simulink model "inner_LQRI_test"  (R2016a)
settings: Solver=VariableStepAuto  StartTime=0.0  StopTime=60  RelTol=1e-3
undefined symbols (not defined in the file or in its folder): b, g, inner_h, inner_maxlim, inner_minlim, K, k, l, m, max_ang_ref
settings Model: Creator=Daniel  LastModifiedBy=mgreiff
settings SolverCC: AlgebraicLoopSolver=LineSearch
settings DataIOCC: LimitDataPoints=on
settings DebuggingCC: AllowSymbolicDim=off
settings ModelReferenceCC: PropagateSignalLabelsOutOfModel=off
settings GRTTargetCC: GeneratePreprocessorConditionals=Use local settings

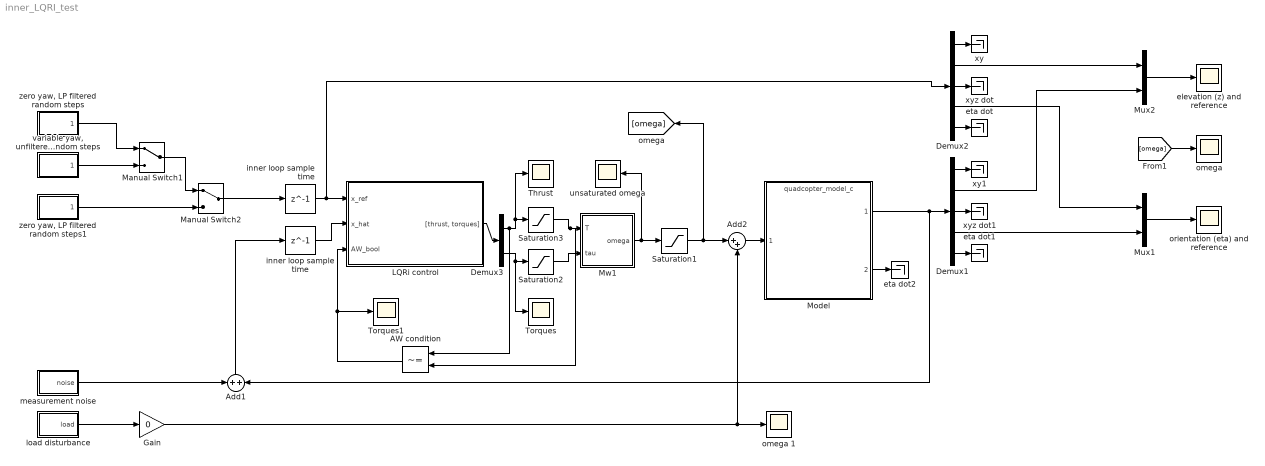
== system inner_LQRI_test ==
  "   eta dot" : Terminator
  "   eta dot1" : Terminator
  "   eta dot2" : Terminator
  "   xy" : Terminator
  "   xy1" : Terminator
  "  xyz dot" : Terminator
  "  xyz dot1" : Terminator
  AW condition : RelationalOperator  Operator=~=  OutDataTypeStr=boolean
  Add1 : Sum
  Add2 : Sum  Inputs=|++
  Demux1 : Demux  Outputs=[2,1,3,3,3]
  Demux2 : Demux  Outputs=[2,1,3,3,3]
  Demux3 : Demux  Outputs=[1,3]
  Gain : Gain  Gain=0
  LQRi control : Subsystem
  Manual Switch1 : ManualSwitch
  Manual Switch2 : ManualSwitch
  Model : ModelReference  ModelNameDialog=quadcopter_model_c.mdl  SimulationMode=Normal  ModelReferenceVersion=1.156
  Mux1 : Mux  Inputs=2
  Mux2 : Mux  Inputs=2
  Mw1 : Subsystem
  Saturation1 : Saturate  UpperLimit=inner_maxlim  LowerLimit=inner_minlim
  Saturation2 : Saturate  UpperLimit=0.1  LowerLimit=-0.1
  Saturation3 : Saturate  LowerLimit=0.01
  Thrust : Scope
  Torques : Scope
  Torques1 : Scope
  elevation (z) and reference : Scope
  inner loop sample time : Delay  DelayLength=1  InitialCondition=0  SampleTime=inner_h
  "inner loop sample time " : Delay  DelayLength=1  InitialCondition=0  SampleTime=inner_h
  load disturbance : Subsystem
  measurement noise : Subsystem
  "omega " : Scope
  omega 1 : Scope
  orientation (eta) and reference : Scope
  unsaturated omega : Scope
  "variable yaw, unfiltered random steps" : Subsystem
  "zero yaw, LP filtered random steps" : Subsystem
  "zero yaw, LP filtered random steps1" : Subsystem
  wires:
  Demux2/2 -> Mux2/1
  Mux2/1 -> elevation (z) and reference/1
  Demux1/2 -> Mux2/2
  Model/1 -> Demux1/1, Add1/2
  Mux1/1 -> orientation (eta) and reference/1
  Saturation1/1 -> [omega], Add2/1
  "inner loop sample time "/1 -> LQRi control/2(x_hat)
  Demux2/3 -> "  xyz dot"/1
  Demux2/5 -> "   eta dot"/1
  Demux2/1 -> "   xy"/1
  Demux1/3 -> "  xyz dot1"/1
  Demux1/5 -> "   eta dot1"/1
  Demux1/1 -> "   xy1"/1
  Demux1/4 -> Mux1/2
  [omega] -> "omega "/1
  Model/2 -> "   eta dot2"/1
  Demux2/4 -> Mux1/1
  AW condition/1 -> Torques1/1, LQRi control/3(AW_bool)
  inner loop sample time/1 -> LQRi control/1(x_ref), Demux2/1
  Manual Switch2/1 -> inner loop sample time/1
  load disturbance/1(load) -> Gain/1
  measurement noise/1(noise) -> Add1/1
  Manual Switch1/1 -> Manual Switch2/1
  Add1/1 -> "inner loop sample time "/1
  Add2/1 -> Model/1
  LQRi control/1("[thrust, torques]") -> Demux3/1
  Demux3/1 -> AW condition/1, Thrust/1, Saturation3/1
  Demux3/2 -> Torques/1, Saturation2/1
  Mw1/1(omega) -> unsaturated omega/1, Saturation1/1
  Saturation2/1 -> Mw1/2(tau)
  Saturation3/1 -> AW condition/2, Mw1/1(T)
  "variable yaw, unfiltered random steps"/1(reference) -> Manual Switch1/2
  "zero yaw, LP filtered random steps"/1(reference) -> Manual Switch1/1
  "zero yaw, LP filtered random steps1"/1(reference) -> Manual Switch2/2
  Gain/1 -> Add2/2, omega 1/1

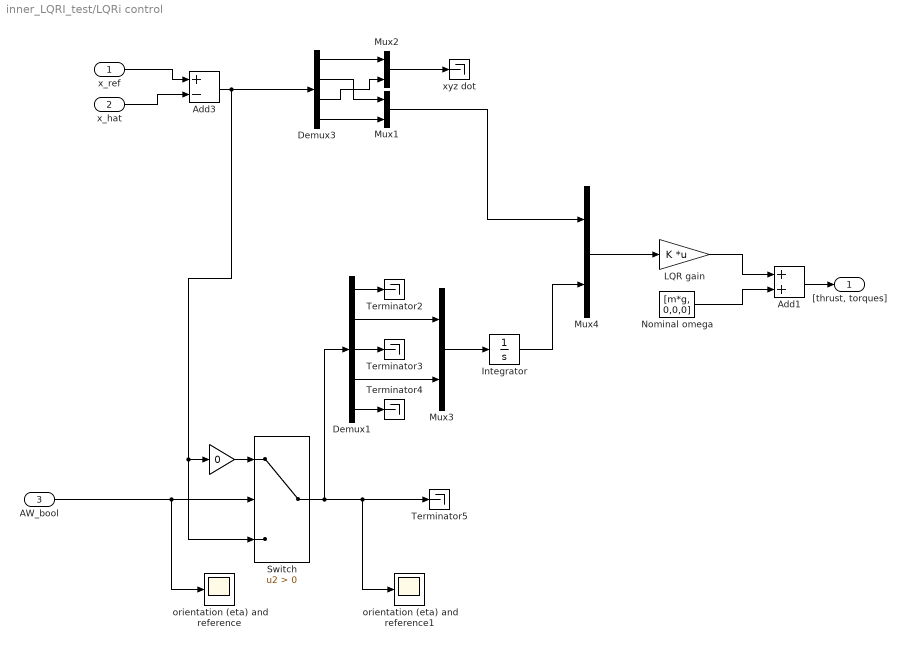
== system inner_LQRI_test/LQRi control ==
  x_ref : Inport  PortDimensions=12
  x_hat : Inport  Port=2  PortDimensions=12
  AW_bool : Inport  Port=3  PortDimensions=1
  "    " : Gain  Gain=0
  "  xyz dot" : Terminator
  Add1 : Sum
  Add3 : Sum  Inputs=+-
  Demux1 : Demux  Outputs=[2,1,3,3,3]
  Demux3 : Demux  Outputs=[2,1,2,7]
  Integrator : Integrator
  LQR gain : Gain  Gain=K  Multiplication=Matrix(K*u)
  Mux{1..4} (4 alike) : Mux  Inputs=2
  Nominal omega : Constant  Value=[m*g, 0,0,0]
  Switch : Switch  Criteria=u2 > Threshold
  Terminator{2..5} (4 alike) : Terminator
  orientation (eta) and reference : Scope
  orientation (eta) and reference1 : Scope
  "[thrust, torques]" : Outport
  wires:
  Mux1/1 -> Mux4/1
  Demux3/4 -> Mux1/2
  Demux3/2 -> Mux1/1
  Demux3/1 -> Mux2/1
  Demux3/3 -> Mux2/2
  Add3/1 -> Switch/3, "    "/1, Demux3/1
  Mux2/1 -> "  xyz dot"/1
  x_ref/1 -> Add3/1
  Demux1/2 -> Mux3/1
  Demux1/3 -> Terminator3/1
  Demux1/4 -> Mux3/2
  Demux1/5 -> Terminator4/1
  Mux3/1 -> Integrator/1
  Integrator/1 -> Mux4/2
  AW_bool/1 -> orientation (eta) and reference/1, Switch/2
  Switch/1 -> Demux1/1, orientation (eta) and reference1/1, Terminator5/1
  "    "/1 -> Switch/1
  LQR gain/1 -> Add1/1
  Nominal omega/1 -> Add1/2
  Add1/1 -> "[thrust, torques]"/1
  Mux4/1 -> LQR gain/1
  Demux1/1 -> Terminator2/1
  x_hat/1 -> Add3/2

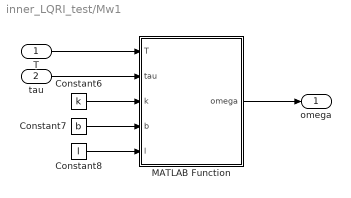
== system inner_LQRI_test/Mw1 ==
  T : Inport
  tau : Inport  Port=2
  Constant6 : Constant  Value=k
  Constant7 : Constant  Value=b
  Constant8 : Constant  Value=l
  MATLAB Function : MATLAB Function  TreatAsAtomicUnit=on
  omega : Outport
  wires:
  Constant7/1 -> MATLAB Function/4(b)
  tau/1 -> MATLAB Function/2(tau)
  Constant6/1 -> MATLAB Function/3(k)
  MATLAB Function/1(omega) -> omega/1
  T/1 -> MATLAB Function/1(T)
  Constant8/1 -> MATLAB Function/5(l)

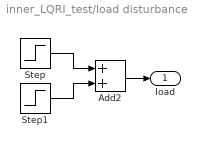
== system inner_LQRI_test/load disturbance ==
  Add2 : Sum
  Step : Step  Time=15  After=500  SampleTime=0
  Step1 : Step  Time=35  After=-500  SampleTime=0
  load : Outport
  wires:
  Add2/1 -> load/1
  Step/1 -> Add2/1
  Step1/1 -> Add2/2

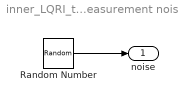
== system inner_LQRI_test/measurement noise ==
  Random Number : RandomNumber  Mean=[0,0,0,0,0,0,0,0,0,0,0,0]  Variance=[0,0,0,0,0,0,0,0,0,0,0,0]
  noise : Outport
  wires:
  Random Number/1 -> noise/1

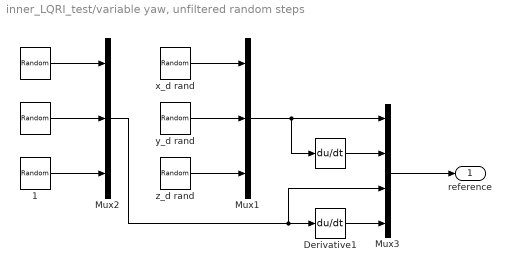
== system inner_LQRI_test/variable yaw, unfiltered random steps ==
  " " : UniformRandomNumber  Minimum=-0.8  Maximum=0.8  Seed=4  SampleTime=10
  "   " : UniformRandomNumber  Minimum=-0.2  Maximum=0.2  Seed=3  SampleTime=10
  "        " : Derivative
  " 1" : UniformRandomNumber  Minimum=-0.8  Maximum=0.8  Seed=5  SampleTime=10
  Derivative1 : Derivative
  Mux1 : Mux  Inputs=3
  Mux2 : Mux  Inputs=3
  Mux3 : Mux  Inputs=[3,3,3,3]
  x_d rand : UniformRandomNumber  Minimum=-30  Maximum=30  SampleTime=10
  y_d rand : UniformRandomNumber  Minimum=-30  Maximum=30  Seed=1  SampleTime=10
  z_d rand : UniformRandomNumber  Minimum=0  Maximum=15  Seed=2  SampleTime=10
  reference : Outport
  wires:
  Mux1/1 -> "        "/1, Mux3/1
  Mux3/1 -> reference/1
  Derivative1/1 -> Mux3/4
  "        "/1 -> Mux3/2
  Mux2/1 -> Mux3/3, Derivative1/1
  "   "/1 -> Mux2/1
  " "/1 -> Mux2/2
  " 1"/1 -> Mux2/3
  x_d rand/1 -> Mux1/1
  y_d rand/1 -> Mux1/2
  z_d rand/1 -> Mux1/3

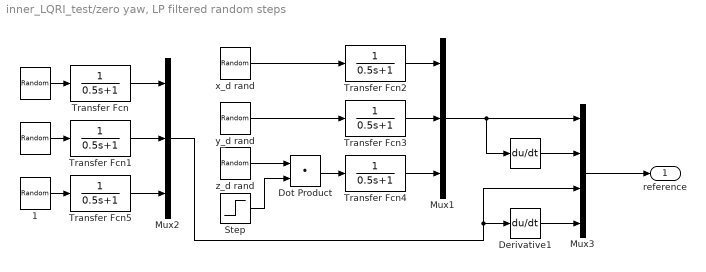
== system inner_LQRI_test/zero yaw, LP filtered random steps ==
  " " : UniformRandomNumber  Minimum=-max_ang_ref  Maximum=max_ang_ref  Seed=4  SampleTime=10
  "   " : UniformRandomNumber  Minimum=-max_ang_ref  Maximum=max_ang_ref  Seed=3  SampleTime=10
  "        " : Derivative
  " 1" : UniformRandomNumber  Minimum=-max_ang_ref  Maximum=max_ang_ref  Seed=5  SampleTime=10
  Derivative1 : Derivative
  Dot Product : DotProduct  InputSameDT=on  OutDataTypeStr=Inherit: Inherit via internal rule
  Mux1 : Mux  Inputs=3
  Mux2 : Mux  Inputs=3
  Mux3 : Mux  Inputs=[3,3,3,3]
  Step : Step  Time=40  Before=1  After=0  SampleTime=0
  Transfer Fcn{,1..5} (6 alike) : TransferFcn  Denominator=[0.5 1]
  x_d rand : UniformRandomNumber  Minimum=-30  Maximum=30  SampleTime=10
  y_d rand : UniformRandomNumber  Minimum=-30  Maximum=30  Seed=1  SampleTime=10
  z_d rand : UniformRandomNumber  Minimum=0  Maximum=3  Seed=2  SampleTime=10
  reference : Outport
  wires:
  Mux1/1 -> "        "/1, Mux3/1
  Mux3/1 -> reference/1
  Derivative1/1 -> Mux3/4
  "        "/1 -> Mux3/2
  Mux2/1 -> Mux3/3, Derivative1/1
  "   "/1 -> Transfer Fcn/1
  " "/1 -> Transfer Fcn1/1
  Transfer Fcn/1 -> Mux2/1
  Transfer Fcn1/1 -> Mux2/2
  Transfer Fcn5/1 -> Mux2/3
  x_d rand/1 -> Transfer Fcn2/1
  y_d rand/1 -> Transfer Fcn3/1
  Transfer Fcn2/1 -> Mux1/1
  Transfer Fcn3/1 -> Mux1/2
  Transfer Fcn4/1 -> Mux1/3
  Step/1 -> Dot Product/2
  z_d rand/1 -> Dot Product/1
  Dot Product/1 -> Transfer Fcn4/1
  " 1"/1 -> Transfer Fcn5/1

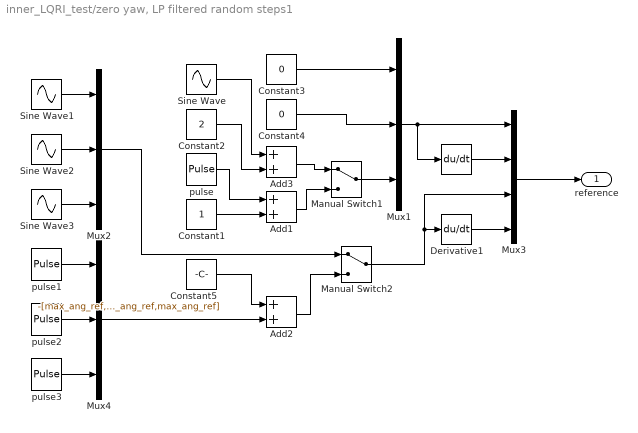
== system inner_LQRI_test/zero yaw, LP filtered random steps1 ==
  "        " : Derivative
  Add1 : Sum
  Add2 : Sum
  Add3 : Sum
  Constant1 : Constant
  Constant2 : Constant  Value=2
  Constant3 : Constant  Value=0
  Constant4 : Constant  Value=0
  Constant5 : Constant  Value=-[max_ang_ref,max_ang_ref,max_ang_ref]
  Derivative1 : Derivative
  Manual Switch1 : ManualSwitch
  Manual Switch2 : ManualSwitch
  Mux1 : Mux  Inputs=3
  Mux2 : Mux  Inputs=3
  Mux3 : Mux  Inputs=[3,3,3,3]
  Mux4 : Mux  Inputs=3
  Sine Wave : Sin  SampleTime=0
  Sine Wave1 : Sin  Amplitude=max_ang_ref  SampleTime=0
  Sine Wave2 : Sin  Amplitude=max_ang_ref  Phase=pi/2
  Sine Wave3 : Sin  Amplitude=max_ang_ref  Phase=pi  SampleTime=0
  pulse : DiscretePulseGenerator  PulseType=Time based  Amplitude=2  Period=10  PulseWidth=50
  pulse1 : DiscretePulseGenerator  PulseType=Time based  Amplitude=max_ang_ref*2  Period=10  PulseWidth=50
  pulse2 : DiscretePulseGenerator  PulseType=Time based  Amplitude=max_ang_ref*2  Period=10  PulseWidth=50
  pulse3 : DiscretePulseGenerator  PulseType=Time based  Amplitude=max_ang_ref*2  Period=10  PulseWidth=50
  reference : Outport
  wires:
  Mux1/1 -> "        "/1, Mux3/1
  Mux3/1 -> reference/1
  Derivative1/1 -> Mux3/4
  "        "/1 -> Mux3/2
  Sine Wave1/1 -> Mux2/1
  Sine Wave2/1 -> Mux2/2
  Sine Wave3/1 -> Mux2/3
  Constant3/1 -> Mux1/1
  Constant4/1 -> Mux1/2
  Sine Wave/1 -> Add3/1
  Constant2/1 -> Add3/2
  Add3/1 -> Manual Switch1/1
  Manual Switch1/1 -> Mux1/3
  Add1/1 -> Manual Switch1/2
  Constant1/1 -> Add1/2
  pulse/1 -> Add1/1
  pulse1/1 -> Mux4/1
  pulse2/1 -> Mux4/2
  pulse3/1 -> Mux4/3
  Constant5/1 -> Add2/1
  Mux4/1 -> Add2/2
  Mux2/1 -> Manual Switch2/1
  Add2/1 -> Manual Switch2/2
  Manual Switch2/1 -> Mux3/3, Derivative1/1

== matlab function inner_LQRI_test/Mw1/MATLAB Function ==
  data: T input; omega output; tau input; k input; b input; l input
function omega = Mw(T, tau, k, b, l)
%#codegen
tau_phi = tau(1);
tau_theta = tau(2);
tau_psi = tau(3);
w1sq = T/(4*k) - tau_theta/(2*k*l) - tau_psi / (4*b);
w2sq = T/(4*k) - tau_phi/(2*k*l) + tau_psi / (4*b);
w3sq = T/(4*k) + tau_theta/(2*k*l) - tau_psi / (4*b);
w4sq = T/(4*k) + tau_phi/(2*k*l) + tau_psi / (4*b);

omega = sqrt(max([w1sq w2sq w3sq w4sq]', 0));
